simulink model "mIKINValidator"  (R2021a)
settings: Solver=VariableStepAuto  StartTime=0.0  StopTime=inf  RelTol=1e-3
values from neighbouring files (symbols this model uses):
  adMotorLimits = [ 0, 180 ... (first row only)    [initSim.m]
  adWeight = [0 0 0 1 1 1]    [initSim.m]    (also in validatorScript.m)
undefined symbols (not defined in the file or in its folder): adA, adAlpha, adD, adHome6rad, adLinkLenghts, adOffset, adWS, Levenberg, Marquardt
libraries: robotcorelib x3, aerolibconvert2 x2, robotmaniplib x2
settings Model: Creator=angelo  LastModifiedBy=angelo

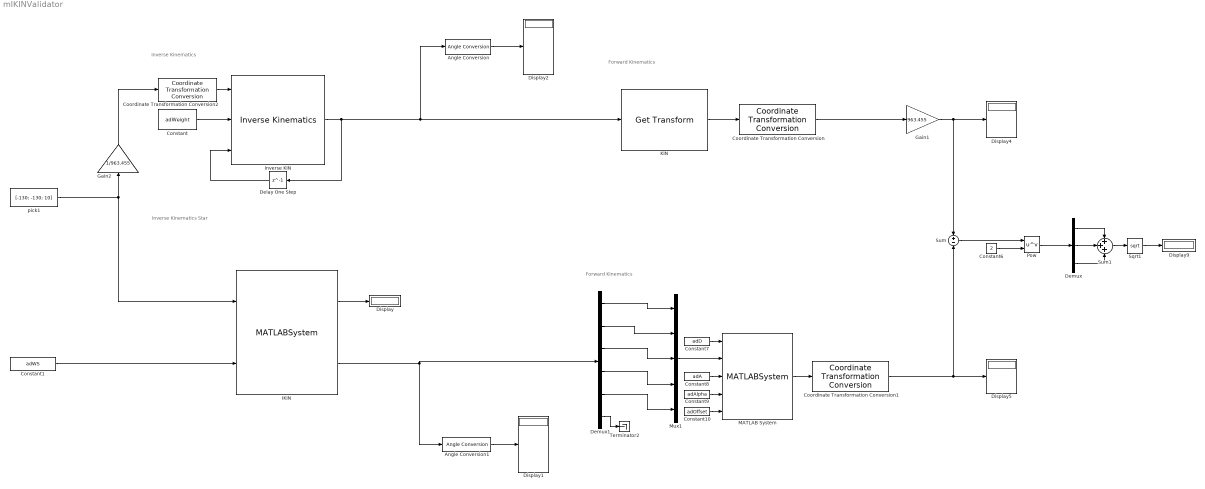
== system mIKINValidator ==
  note: Inverse Kinematics
  note: Inverse Kinematics Star
  note: Forward Kinematics
  note: Forward Kinematics
  Angle Conversion : aerolibconvert2/Angle Conversion  IU=rad  OU=deg
  Angle Conversion1 : aerolibconvert2/Angle Conversion  IU=rad  OU=deg
  Constant : Constant  Value=adWeight
  Constant1 : Constant  Value=adWS
  Constant10 : Constant  Value=adOffset
  Constant6 : Constant  Value=2
  Constant7 : Constant  Value=adD
  Constant8 : Constant  Value=adA
  Constant9 : Constant  Value=adAlpha
  Coordinate Transformation Conversion : robotcorelib/Coordinate Transformation Conversion  InputRepresentation=Homogeneous Transformation  InputEulerSequence=ZYX  ShowTrVecInputPort=on  OutputRepresentation=Translation Vector  OutputEulerSequence=ZYX  ShowTrVecOutputPort=on  SimulateUsing=Interpreted execution
      settings: SourceProductBaseCode=NV,RO,RR,UV
  Coordinate Transformation Conversion1 : robotcorelib/Coordinate Transformation Conversion  InputRepresentation=Homogeneous Transformation  InputEulerSequence=ZYX  ShowTrVecInputPort=on  OutputRepresentation=Translation Vector  OutputEulerSequence=ZYX  ShowTrVecOutputPort=on  SimulateUsing=Interpreted execution
      settings: SourceProductBaseCode=NV,RO,RR,UV
  Coordinate Transformation Conversion2 : robotcorelib/Coordinate Transformation Conversion  InputRepresentation=Translation Vector  InputEulerSequence=ZYX  ShowTrVecInputPort=on  OutputRepresentation=Homogeneous Transformation  OutputEulerSequence=ZYX  ShowTrVecOutputPort=on  SimulateUsing=Interpreted execution
      settings: SourceProductBaseCode=NV,RO,RR,UV
  Delay One Step : Delay  DelayLength=1  InitialCondition=adHome6rad
  Demux : Demux  Outputs=3
  Demux1 : Demux  Outputs=6
  Display{,1..2,4..5,9} (6 alike) : Display
  Gain1 : Gain  Gain=963.455
  Gain2 : Gain  Gain=1/963.455
  IKIN : MATLABSystem  System=oIKINSolver  adHomeDeg=adHome6deg  nGroundLength=adLinkLenghts(1)  nArmLength=adLinkLenghts(2)  nForearmLength=adLinkLenghts(3)  nHandLength=adLinkLenghts(4)  adBaseMinMaxDeg=adMotorLimits(1,:)  adShoulderMinMaxDeg=adMotorLimits(2,:)  adElbowMinMaxDeg=adMotorLimits(3,:)  adPitchMinMaxDeg=adMotorLimits(4,:)  adRollMinMaxDeg=adMotorLimits(5,:)  SimulateUsing=Code generation
      mask Type: oIKINSolver
      mask Display:
      | disp('oIKINSolver');
      | port_label('input',1,'adPoint');
      | port_label('input',2,'adWS');
      | port_label('output',1,'bFlag');
      | port_label('output',2,'adJC');
  Inverse KIN : robotmaniplib/Inverse Kinematics  RigidBodyTree=oBraccio6dofee  EndEffector=ee  ShowInfo=off  SolverName=Levenberg-Marquardt  EnforceJointLimits=on  MaxIterations=1500  MaxTime=10  GradientTolerance=1e-7  SolutionTolerance=1e-6  StepTolerance=1e-14  ErrorChangeTolerance=1e-12  UseErrorDamping=on  DampingBias=0.0025  SimulateUsing=Interpreted execution
  KIN : robotmaniplib/Get Transform  RigidBodyTree=oBraccio6dofee  SourceBody=ee  TargetBody=base_link  SimulateUsing=Interpreted execution
  MATLAB System : MATLABSystem  System=oKINSolver  adHomeDeg=adHome6deg  nGroundLength=adLinkLenghts(1)  nArmLength=adLinkLenghts(2)  nForearmLength=adLinkLenghts(3)  nHandLength=adLinkLenghts(4)  adBaseMinMaxDeg=adMotorLimits(1,:)  adShoulderMinMaxDeg=adMotorLimits(2,:)  adElbowMinMaxDeg=adMotorLimits(3,:)  adPitchMinMaxDeg=adMotorLimits(4,:)  adRollMinMaxDeg=adMotorLimits(5,:)  SimulateUsing=Code generation
      mask Type: oKINSolver
      mask Display:
      | disp('oKINSolver');
      | port_label('input',1,'adD');
      | port_label('input',2,'adQ');
      | port_label('input',3,'adA');
      | port_label('input',4,'adAlpha');
      | port_label('input',5,'adOffset');
      | port_label('output',1,'adPoint');
  Mux1 : Mux  Inputs=5
  Pow : Math  Operator=pow  RndMeth=Zero  SaturateOnIntegerOverflow=on
  Sqrt1 : Sqrt  SaturateOnIntegerOverflow=on
  Sum : Sum  Inputs=+|-
  Sum1 : Sum  Inputs=+++
  Terminator2 : Terminator
  pick1 : Constant  Value=[-130; -130; 10]
  wires:
  Constant/1 -> Inverse KIN/2
  Delay One Step/1 -> Inverse KIN/3
  Inverse KIN/1 -> Angle Conversion/1, KIN/1, Delay One Step/1
  Coordinate Transformation Conversion2/1 -> Inverse KIN/1
  IKIN/2 -> Angle Conversion1/1, Demux1/1
  Constant1/1 -> IKIN/2
  IKIN/1 -> Display/1
  Angle Conversion1/1 -> Display1/1
  KIN/1 -> Coordinate Transformation Conversion/1
  Demux1/6 -> Terminator2/1
  Demux1/5 -> Mux1/5
  Demux1/2 -> Mux1/2
  Mux1/1 -> MATLAB System/2
  Demux1/3 -> Mux1/3
  Demux1/1 -> Mux1/1
  Demux1/4 -> Mux1/4
  Coordinate Transformation Conversion1/1 -> Sum/2, Display5/1
  Coordinate Transformation Conversion/1 -> Gain1/1
  Gain2/1 -> Coordinate Transformation Conversion2/1
  Gain1/1 -> Display4/1, Sum/1
  Angle Conversion/1 -> Display2/1
  pick1/1 -> IKIN/1, Gain2/1
  Demux/2 -> Sum1/2
  Demux/1 -> Sum1/1
  Demux/3 -> Sum1/3
  Sum/1 -> Pow/1
  Pow/1 -> Demux/1
  Sum1/1 -> Sqrt1/1
  Sqrt1/1 -> Display9/1
  Constant6/1 -> Pow/2
  Constant10/1 -> MATLAB System/5
  Constant8/1 -> MATLAB System/3
  Constant9/1 -> MATLAB System/4
  Constant7/1 -> MATLAB System/1
  MATLAB System/1 -> Coordinate Transformation Conversion1/1
